simulink model "Water_Supply_Network"  (R2024a)
settings: Solver=VariableStepAuto  StartTime=0.0  StopTime=10.0  RelTol=1e-3
model workspace (MAT data in the model file):
  a_1 = Simulink.Parameter
  a_1.Complexity = 'real'
  a_1.Dimensions = [0 0]
  a_1.DataType = 'auto'
  c1 = Simulink.Parameter
  c1.Complexity = 'real'
  c1.Dimensions = [0 0]
  c1.DataType = 'auto'
  c1_init = Simulink.Parameter
  c1_init.Complexity = 'real'
  c1_init.Dimensions = [0 0]
  c1_init.DataType = 'auto'
  ci_init = 1
  d_1 = Simulink.Parameter
  d_1.Complexity = 'real'
  d_1.Dimensions = [0 0]
  d_1.DataType = 'auto'
  f_1 = Simulink.Parameter
  f_1.Complexity = 'real'
  f_1.Dimensions = [0 0]
  f_1.DataType = 'auto'
  p1 = Simulink.Parameter
  p1.Complexity = 'real'
  p1.Dimensions = [0 0]
  p1.DataType = 'auto'
settings Model: Creator=Anna  LastModifiedBy=Anna

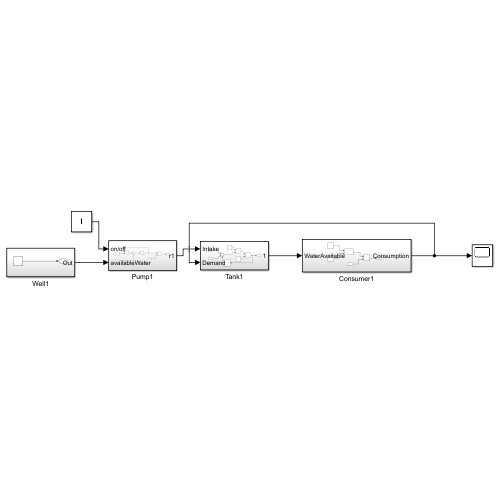
[thumbnail: Simulink's stored preview of the top-level diagram]
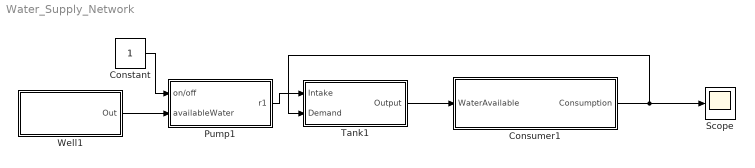
== system Water_Supply_Network ==
  Constant : Constant
  Consumer1 : Subsystem
  Pump1 : Subsystem
  Scope : Scope
  Tank1 : Subsystem
  Well1 : Subsystem
  wires:
  Well1/1(Out) -> Pump1/2(availableWater)
  Tank1/1(Output) -> Consumer1/1(WaterAvailable)
  Consumer1/1(Consumption) -> Scope/1, Tank1/2(Demand)
  Pump1/1(r1) -> Tank1/1(Intake)
  Constant/1 -> Pump1/1(on/off)

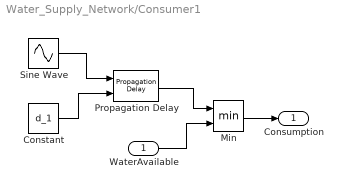
== system Water_Supply_Network/Consumer1 ==
  WaterAvailable : Inport
  Constant : Constant  Value=d_1
  Min : MinMax  Inputs=2
  Propagation Delay : PropagationDelay  InitialOutput=a_1
  Sine Wave : Sin  Amplitude=a_1  Bias=a_1  Frequency=f_1  SampleTime=0
  Consumption : Outport
  wires:
  Sine Wave/1 -> Propagation Delay/1
  Constant/1 -> Propagation Delay/2
  WaterAvailable/1 -> Min/2
  Min/1 -> Consumption/1
  Propagation Delay/1 -> Min/1

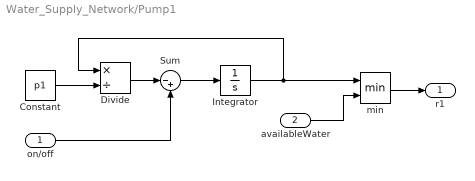
== system Water_Supply_Network/Pump1 ==
  on/off : Inport  OutDataTypeStr=boolean
  availableWater : Inport  Port=2
  Constant : Constant  Value=p1
  Divide : Product  Inputs=*/
  Integrator : Integrator
  Sum : Sum  Inputs=|-+
  min : MinMax  Inputs=2
  r1 : Outport
  wires:
  on/off/1 -> Sum/2
  Sum/1 -> Integrator/1
  Integrator/1 -> Divide/1, min/1
  Constant/1 -> Divide/2
  Divide/1 -> Sum/1
  availableWater/1 -> min/2
  min/1 -> r1/1

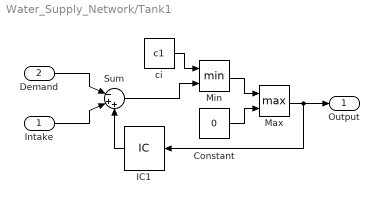
== system Water_Supply_Network/Tank1 ==
  Intake : Inport
  Demand : Inport  Port=2
  Constant : Constant  Value=0
  IC1 : InitialCondition  Value=c1_init
  Max : MinMax  Function=max  Inputs=2
  Min : MinMax  Inputs=2
  Sum : Sum  Inputs=|-++
  ci : Constant  Value=c1
  Output : Outport
  wires:
  Intake/1 -> Sum/2
  Sum/1 -> Min/2
  ci/1 -> Min/1
  Demand/1 -> Sum/1
  IC1/1 -> Sum/3
  Min/1 -> Max/1
  Constant/1 -> Max/2
  Max/1 -> IC1/1, Output/1

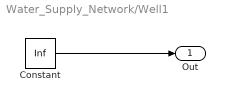
== system Water_Supply_Network/Well1 ==
  Constant : Constant  Value=Inf
  Out : Outport
  wires:
  Constant/1 -> Out/1
